simulink model "Cascade0"  (R2020a)
settings: Solver=FixedStepAuto  StartTime=0.0  StopTime=10.0  FixedStep=0.2  RelTol=1e-3
settings Model: Creator=Shivam  LastModifiedBy=Shivam
settings DataIOCC: SaveOutput=off  SaveTime=off

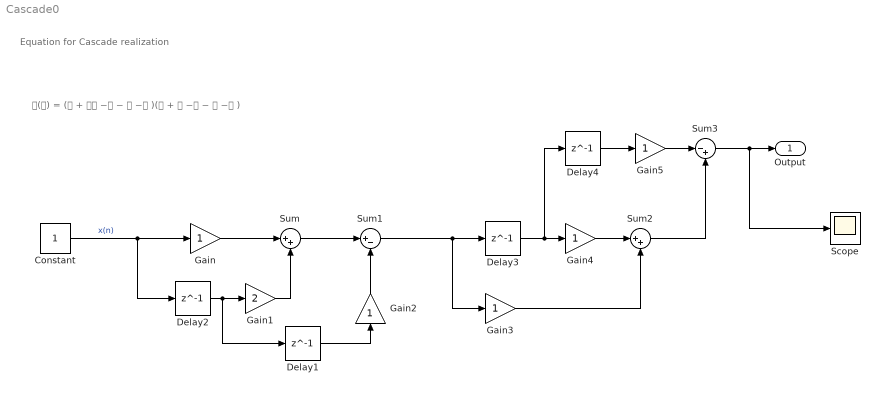
== system Cascade0 ==
  note: 𝐇(𝐳) = (𝟏 + 𝟐𝐳 −𝟏 − 𝐳 −𝟐 )(𝟏 + 𝐳 −𝟏 − 𝐳 −𝟐 )
  note: Equation for Cascade realization
  Constant : Constant
  Delay{1..4} (4 alike) : Delay  DelayLength=1
  Gain{,2..5} (5 alike) : Gain
  Gain1 : Gain  Gain=2
  Scope : Scope
  Sum : Sum  Inputs=|++
  Sum1 : Sum  Inputs=|+-
  Sum2 : Sum  Inputs=|++
  Sum3 : Sum  Inputs=|-+
  Output : Outport  OutDataTypeStr=double  PortDimensions=1  SampleTime=[0.20000000000000001,0]
  wires:
  Delay1/1 -> Gain2/1
  Sum1/1 -> Delay3/1, Gain3/1
  Constant/1 -> Delay2/1, Gain/1  "x(n)"
  Gain/1 -> Sum/1
  Sum3/1 -> Scope/1, Output/1
  Delay3/1 -> Gain4/1, Delay4/1
  Sum/1 -> Sum1/1
  Delay2/1 -> Gain1/1, Delay1/1
  Gain5/1 -> Sum3/1
  Delay4/1 -> Gain5/1
  Gain4/1 -> Sum2/1
  Gain2/1 -> Sum1/2
  Gain3/1 -> Sum2/2
  Sum2/1 -> Sum3/2
  Gain1/1 -> Sum/2
